simulink model "motor_base"  (R2019b)
settings: Solver=VariableStepAuto  StartTime=0.0  StopTime=10.0  RelTol=1e-3
libraries: cstblocks x10
settings Model: Creator=Dell  LastModifiedBy=Dell

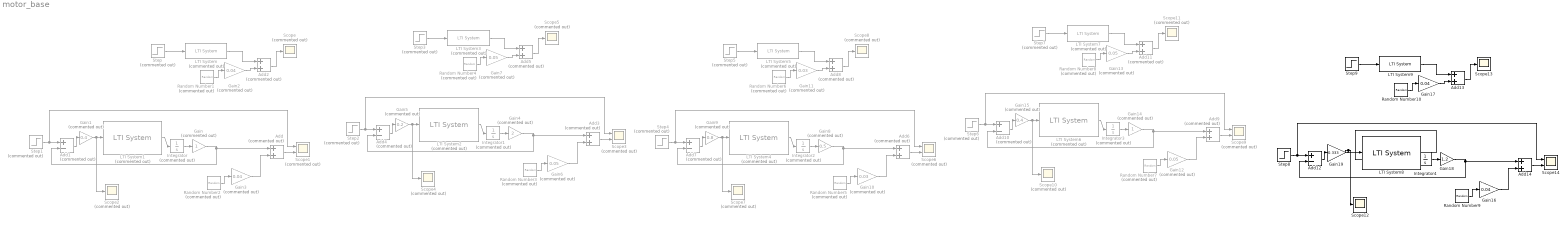
== system motor_base ==
  Add{,2..3,5..6,8..9,11} (8 alike) : Sum  Commented=on
  Add{1,4,7,10} (4 alike) : Sum  Commented=on  Inputs=+-
  Add12 : Sum  Inputs=+-
  Add13 : Sum
  Add14 : Sum
  Gain : Gain  Commented=on
  Gain1 : Gain  Commented=on  Gain=0.4
  Gain10 : Gain  Commented=on  Gain=0.03
  Gain11 : Gain  Commented=on  Gain=0.03
  Gain{6..7,12..13} (4 alike) : Gain  Commented=on  Gain=0.05
  Gain14 : Gain  Commented=on
  Gain15 : Gain  Commented=on  Gain=0.4
  Gain16 : Gain  Gain=0.04
  Gain17 : Gain  Gain=0.04
  Gain18 : Gain  Gain=1.2
  Gain19 : Gain  Gain=0.333
  Gain2 : Gain  Commented=on  Gain=0.04
  Gain3 : Gain  Commented=on  Gain=0.04
  Gain4 : Gain  Commented=on  Gain=2
  Gain5 : Gain  Commented=on  Gain=0.2
  Gain8 : Gain  Commented=on  Gain=0.5
  Gain9 : Gain  Commented=on  Gain=0.8
  Integrator{,1..3} (4 alike) : Integrator  Commented=on
  Integrator4 : Integrator
  LTI System{,1..7} (8 alike) : cstblocks/LTI System  Commented=on  sys=tf(22.846,[1 3.023 9.139])  IC=[]
  LTI System8 : cstblocks/LTI System  sys=tf(22.846,[1 3.023 9.139])  IC=[]
  LTI System9 : cstblocks/LTI System  sys=tf(22.846,[1 3.023 9.139])  IC=[]
  Random Number{1..8} (8 alike) : RandomNumber  Commented=on  SampleTime=0.01
  Random Number10 : RandomNumber  SampleTime=0.01
  Random Number9 : RandomNumber  SampleTime=0.01
  Scope{,2,4..5,7..8,10..11} (8 alike) : Scope  Commented=on
  Scope{1,3,6,9} (4 alike) : Scope  Commented=on  NumInputPorts=2
  Scope12 : Scope
  Scope13 : Scope
  Scope14 : Scope  NumInputPorts=2
  Step : Step  Commented=on  Time=0  After=randi(200)  SampleTime=0
  Step1 : Step  Commented=on  Time=0  After=randi(200)  SampleTime=0
  Step2 : Step  Commented=on  Time=0  After=randi(250)  SampleTime=0
  Step3 : Step  Commented=on  Time=0  After=randi(250)  SampleTime=0
  Step{4..7} (4 alike) : Step  Commented=on  Time=0  After=randi(40)  SampleTime=0
  Step8 : Step  Time=0  After=randi(40)  SampleTime=0
  Step9 : Step  Time=0  After=randi(40)  SampleTime=0
  wires:
  Step/1 -> LTI System/1
  Step1/1 -> Scope1/1, Add1/1
  LTI System1/1 -> Integrator/1
  Integrator/1 -> Gain/1
  Gain/1 -> Add1/2, Add/1
  Gain1/1 -> Scope2/1, LTI System1/1
  Add1/1 -> Gain1/1
  Add/1 -> Scope1/2
  Gain3/1 -> Add/2
  Add2/1 -> Scope/1
  LTI System/1 -> Add2/1
  Gain2/1 -> Add2/2
  Random Number1/1 -> Gain2/1
  Random Number2/1 -> Gain3/1
  Random Number3/1 -> Gain6/1
  Gain5/1 -> Scope4/1, LTI System2/1
  Gain4/1 -> Add4/2, Add3/1
  Add4/1 -> Gain5/1
  Integrator1/1 -> Gain4/1
  LTI System2/1 -> Integrator1/1
  Step2/1 -> Scope3/1, Add4/1
  Add3/1 -> Scope3/2
  Add5/1 -> Scope5/1
  Random Number4/1 -> Gain7/1
  LTI System3/1 -> Add5/1
  Step3/1 -> LTI System3/1
  Gain7/1 -> Add5/2
  Gain6/1 -> Add3/2
  Step4/1 -> Scope6/1, Add7/1
  LTI System4/1 -> Integrator2/1
  Gain11/1 -> Add8/2
  Step5/1 -> LTI System5/1
  LTI System5/1 -> Add8/1
  Random Number6/1 -> Gain11/1
  Add6/1 -> Scope6/2
  Add8/1 -> Scope8/1
  Gain8/1 -> Add7/2, Add6/1
  Gain9/1 -> Scope7/1, LTI System4/1
  Random Number5/1 -> Gain10/1
  Integrator2/1 -> Gain8/1
  Add7/1 -> Gain9/1
  Gain10/1 -> Add6/2
  Add9/1 -> Scope9/2
  Random Number8/1 -> Gain13/1
  LTI System7/1 -> Add11/1
  Step7/1 -> LTI System7/1
  Gain13/1 -> Add11/2
  Step6/1 -> Scope9/1, Add10/1
  LTI System6/1 -> Integrator3/1
  Add11/1 -> Scope11/1
  Gain12/1 -> Add9/2
  Add10/1 -> Gain15/1
  Gain15/1 -> Scope10/1, LTI System6/1
  Gain14/1 -> Add10/2, Add9/1
  Integrator3/1 -> Gain14/1
  Random Number7/1 -> Gain12/1
  Integrator4/1 -> Gain18/1
  Gain18/1 -> Add12/2, Add14/1
  Random Number9/1 -> Gain16/1
  Add12/1 -> Gain19/1
  Gain16/1 -> Add14/2
  Add13/1 -> Scope13/1
  LTI System8/1 -> Integrator4/1
  Step8/1 -> Scope14/1, Add12/1
  Gain17/1 -> Add13/2
  Random Number10/1 -> Gain17/1
  Step9/1 -> LTI System9/1
  LTI System9/1 -> Add13/1
  Add14/1 -> Scope14/2
  Gain19/1 -> LTI System8/1, Scope12/1
